simulink model "sftry"  (Simulink 7.8)
settings: Solver=ode45  StartTime=0.0  StopTime=10.0  RelTol=1e-3
settings Model: Creator=Birdman  LastModifiedBy=Birdman

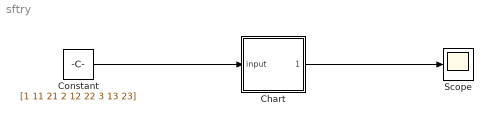
== system sftry ==
  Chart : Stateflow chart  TreatAsAtomicUnit=on
  Constant : Constant  Value=[1 11 21 2 12 22 3 13 23]
  Scope : Scope
  wires:
  Constant/1 -> Chart/1(input)
  Chart/1(output) -> Scope/1

== stateflow chart Chart ==
  state calculation
    en:i=0;
    du:data_info=readdata(input);i++;
  state calculation1
    en:output=data_info;
    du:output=output+1;i=0;
  (default) -> calculation
  calculation -> calculation1 : [i==3]
  calculation1 -> calculation : [i==0]
  data: u function_input double size=9; rd function_output double size=3 =[0 0 0]; input input double; data_info local double size=3; output output double; i local double
  function rd=readdata(u):
    | function rd=readdata(u)
    | rd=zeros(1,3)';
    | rd(1)=u(1);
    | rd(2)=u(2);
    | rd(3)=u(3);
